simulink model "LazoCerrado"  (R2022a)
settings: Solver=VariableStepAuto  StartTime=0.0  StopTime=10.0  RelTol=1e-3
undefined symbols (not defined in the file): x
settings Model: Creator=ec0822  LastModifiedBy=ec0822

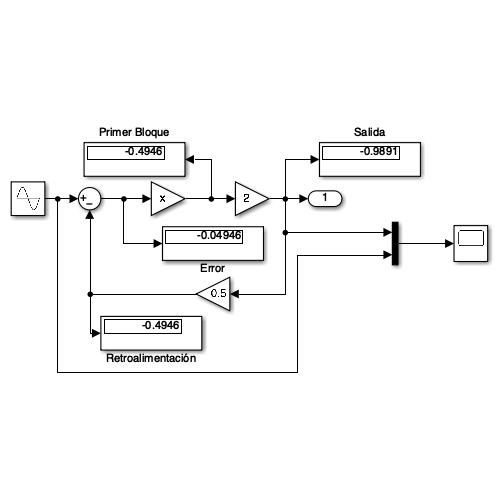
[thumbnail: Simulink's stored preview of the top-level diagram]
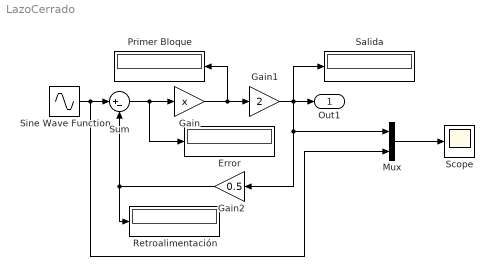
== system LazoCerrado ==
  Error : Display
  Gain : Gain  Gain=x
  Gain1 : Gain  Gain=2
  Gain2 : Gain  Gain=0.5
  Mux : Mux  Inputs=2
  Primer Bloque : Display
  Retroalimentación : Display
  Salida : Display
  Scope : Scope
  Sine Wave Function : Sin  SampleTime=0
  Sum : Sum  Inputs=|+-
  Out1 : Outport
  wires:
  Gain/1 -> Gain1/1, Primer Bloque/1
  Gain1/1 -> Salida/1, Out1/1, Mux/1, Gain2/1
  Gain2/1 -> Sum/2, Retroalimentación/1
  Sum/1 -> Error/1, Gain/1
  Sine Wave Function/1 -> Mux/2, Sum/1
  Mux/1 -> Scope/1
